simulink model "predictorSmith"  (R2015a)
settings: Solver=ode45  StartTime=0.0  StopTime=300  RelTol=1e-3
values from neighbouring files (symbols this model uses):
  D = [1 8.9718032673 37.5635184713 89.8699994005 120.944393138 72.3392867678]    [DatosPF.mat]
  N = [-1 8.9718032673 -37.5635184713 89.8699994005 -120.944393138 72.3392867678]    [DatosPF.mat]
undefined symbols (not defined in the file or in its folder): DD, Dr, NN, Nr
libraries: simulink x1
settings Model: Creator=ADM  LastModifiedBy=ADM

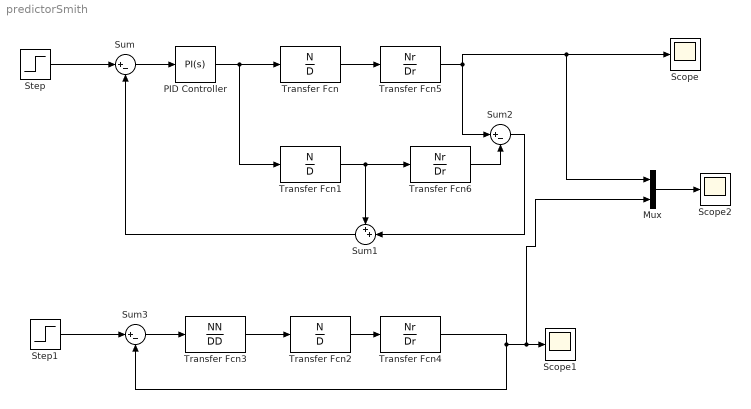
== system predictorSmith ==
  Mux : Mux  Inputs=2
  PID Controller : simulink/Continuous/PID Controller  Controller=PI  TimeDomain=Continuous-time  SampleTime=-1  IntegratorMethod=Forward Euler  FilterMethod=Forward Euler  Form=Parallel  UseFilter=on  ControllerParametersSource=internal  P=1.68363538710378  I=0.113189043355807  D=0  N=100  InitialConditionSource=internal  InitialConditionForIntegrator=0  InitialConditionForFilter=0  ExternalReset=none  LimitOutput=off  UpperSaturationLimit=inf  LowerSaturationLimit=-inf  LinearizeAsGain=on  AntiWindupMode=none  Kb=1  TrackingMode=off  Kt=1  PParamMin=[]  PParamMax=[]  IParamMin=[]  IParamMax=[]  DParamMin=[]  DParamMax=[]  NParamMin=[]  NParamMax=[]  KbParamMin=[]  KbParamMax=[]  KtParamMin=[]  KtParamMax=[]  POutMin=[]  POutMax=[]  IOutMin=[]  IOutMax=[]  DOutMin=[]  DOutMax=[]  NOutMin=[]  NOutMax=[]  KbOutMin=[]  KbOutMax=[]  KtOutMin=[]  KtOutMax=[]  IntegratorOutMin=[]  IntegratorOutMax=[]  FilterOutMin=[]  FilterOutMax=[]  SumOutMin=[]  SumOutMax=[]  SumI1OutMin=[]  SumI1OutMax=[]  SumI2OutMin=[]  SumI2OutMax=[]  SumI3OutMin=[]  SumI3OutMax=[]  SumDOutMin=[]  SumDOutMax=[]  SaturationOutMin=[]  SaturationOutMax=[]  IntegratorContinuousStateAttributes=''  IntegratorStateMustResolveToSignalObject=off  IntegratorRTWStateStorageClass=Auto  FilterContinuousStateAttributes=''  FilterStateMustResolveToSignalObject=off  FilterRTWStateStorageClass=Auto  DifferentiatorICPrevScaledInput=0  DifferentiatorOutMin=[]  DifferentiatorOutMax=[]
  Scope : Scope
  Scope1 : Scope
  Scope2 : Scope
      settings: SaveName=ScopeData2
  Step : Step  SampleTime=0
  Step1 : Step  SampleTime=0
  Sum : Sum  Inputs=|+-
  Sum1 : Sum  Inputs=++|
  Sum2 : Sum  Inputs=|+-
  Sum3 : Sum  Inputs=|+-
  Transfer Fcn : TransferFcn  Numerator=N  Denominator=D
  Transfer Fcn1 : TransferFcn  Numerator=N  Denominator=D
  Transfer Fcn2 : TransferFcn  Numerator=N  Denominator=D
  Transfer Fcn3 : TransferFcn  Numerator=NN  Denominator=DD
  Transfer Fcn4 : TransferFcn  Numerator=Nr  Denominator=Dr
  Transfer Fcn5 : TransferFcn  Numerator=Nr  Denominator=Dr
  Transfer Fcn6 : TransferFcn  Numerator=Nr  Denominator=Dr
  wires:
  Sum/1 -> PID Controller/1
  Transfer Fcn/1 -> Transfer Fcn5/1
  Step/1 -> Sum/1
  PID Controller/1 -> Transfer Fcn1/1, Transfer Fcn/1
  Transfer Fcn5/1 -> Sum2/1, Mux/1, Scope/1
  Transfer Fcn1/1 -> Transfer Fcn6/1, Sum1/1
  Sum2/1 -> Sum1/2
  Sum1/1 -> Sum/2
  Sum3/1 -> Transfer Fcn3/1
  Step1/1 -> Sum3/1
  Transfer Fcn3/1 -> Transfer Fcn2/1
  Transfer Fcn2/1 -> Transfer Fcn4/1
  Transfer Fcn4/1 -> Sum3/2, Mux/2, Scope1/1
  Mux/1 -> Scope2/1
  Transfer Fcn6/1 -> Sum2/2
